simulink model "sampleModel1886"  (R2023a)
settings: Solver=VariableStepAuto  StartTime=0.0  StopTime=10.0  RelTol=1e-3
libraries: hdlsllib x5, simulink x1
settings Model: Creator=user1  LastModifiedBy=user1

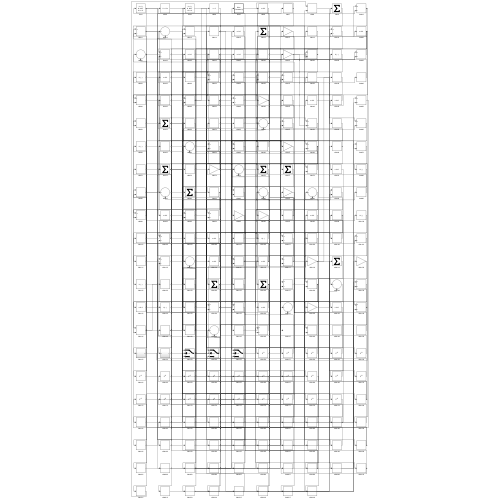
[thumbnail: Simulink's stored preview of the top-level diagram]
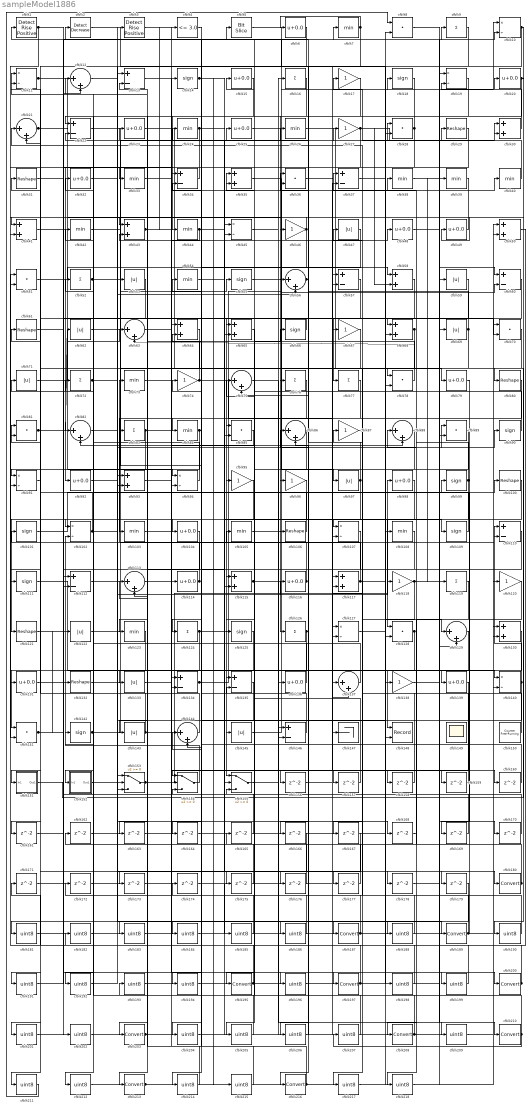
== system sampleModel1886 ==
  cfblk1 : hdlsllib/Logic and Bit Operations/Detect Rise Positive  vinit=0  OutDataTypeStr=boolean
  cfblk{10..11,19,45,91,94,102,107,127,140} (10 alike) : Product  Inputs=*/  RndMeth=Zero  SaturateOnIntegerOverflow=on
  cfblk{29,31,61,80,100,106,121,132} (8 alike) : Reshape
  cfblk{14,18,55,66,90,99,101,109,111,125,142} (11 alike) : Signum
  cfblk{7,24,26,33,38..40,42,44,54,73,84,103,105,108,123} (16 alike) : MinMax
  cfblk{6,15,20,23,25,32,48..49,79,92,98,104,114,116,131,136,139} (17 alike) : Bias  Bias=0.0  SaturateOnIntegerOverflow=off
  cfblk{13,22,34,37,57,60,110,112,134..135,146} (11 alike) : Sum  Inputs=+-
  cfblk{12,21,56,63,75,82,86,88,113,129,137,144} (12 alike) : Sum  Inputs=|++
  cfblk{30,35,41,43,50,58,64..65,68,93,115,117,130} (13 alike) : Sum
  cfblk{17,27,46,67,74,87,95..96,118,120,138} (11 alike) : Gain
  cfblk{9,16,52,72,76..77,83,119,124,126} (10 alike) : Sum  Inputs=+
  cfblk{47,53,59,62,69,71,97,122,133,143,145} (11 alike) : Abs  SaturateOnIntegerOverflow=off
  cfblk{8,28,36,51,70,78,81,85,89,128,141} (11 alike) : DotProduct  OutDataTypeStr=Inherit: Inherit via internal rule
  cfblk147 : Terminator
  cfblk148 : Record  FileSettingsInternal="{\"entries\":[{\"content\":{\"excelSettings\":{\"content\":{},\"type\":\"Streamout.ExcelSettings\"}},\"type\":\"Streamout.FileSettingStorage\",\"uuid\":\"\"}],\"packageUris\":[\"http:\\/\\/schema.mathworks.com\\/mf0\\/streamout_blocks\\/R2020a\"],\"version\":\"1.0\"}"  Layout=[1 1]  SignalsInternal="{\"entries\":[{\"content\":{\"signals\":[{\"content\":{\"blockPath\":[],\"dimensions\":[1],\"domain\":\"\",\"lineColor\":\"#a2142f\",\"plots\":[1],\"port\":1,\"signalID\":4786,\"signalName\":\"XY Graph:1\"},\"type\":\"RecordBlkView.Signal\",\"uuid\":\"\"},{\"content\":{\"blockPath\":[],\"dimensions\":[1],\"domain\":\"\",\"lineColor\":\"#139fff\",\"plots\":[1],\"port\":2,\"signalID\":4789,\"signalName\":\"XY Graph:2\"},\"type\":\"RecordBlkView.Signal\",\"uuid\":\"\"}]},\"type\":\"RecordBlkView.InputSignals\",\"uuid\":\"\"}],\"packageUris\":[\"http:\\/\\/schema.mathworks.com\\/mf0\\/streamout_blocks\\/R2020a\"],\"version\":\"1.0\"}"  VisualizationBindings="{\"xyplotplugin\":{\"info\":[{\"series\":[{\"bindingParametersList\":[{\"parameter\":\"X-Axis\",\"signalID\":4786,\"signalName\":\"XY Graph:1\"},{\"parameter\":\"Y-Axis\",\"signalID\":4789,\"signalName\":\"XY Graph:2\"}],\"seriesID\":2000}],\"subplotID\":1}]}}"  CompatibilityTag=XY  st=-1
  cfblk149 : Scope
      settings: Floating=on
  cfblk150 : hdlsllib/Sources/Counter Free-Running  NumBits=16  tsamp=-1
  cfblk151 : Subsystem
      settings: LibrarySourceBlock=|
      | hdlsllib/Ports &
      | Subsystems/Subsystem
  cfblk152 : Subsystem
      settings: LibrarySourceBlock=|
      | hdlsllib/Ports &
      | Subsystems/Subsystem
  cfblk153 : Switch  SaturateOnIntegerOverflow=off  InputSameDT=off
  cfblk154 : Switch  SaturateOnIntegerOverflow=off  InputSameDT=off
  cfblk155 : Switch  SaturateOnIntegerOverflow=off  InputSameDT=off
  cfblk{156..179} (24 alike) : Delay  SampleTime=1
  cfblk{180,187,189,195,197,200,203,208,210,213,216} (11 alike) : DataTypeConversion  SaturateOnIntegerOverflow=off  RndMeth=Floor
  cfblk{181..186,188,190..194,196,198..199,201..202,204..207,209,211..212,214..215,217..218} (28 alike) : DataTypeConversion  OutDataTypeStr=uint8  SaturateOnIntegerOverflow=off  RndMeth=Floor
  cfblk2 : simulink/Logic and Bit Operations/Detect Decrease  vinit=0.0  OutDataTypeStr=boolean
      settings: LibrarySourceBlock=|
      | hdlsllib/Logic and Bit
      | Operations/Detect
      | Decrease
  cfblk3 : hdlsllib/Logic and Bit Operations/Detect Rise Positive  vinit=0  OutDataTypeStr=boolean
  cfblk4 : hdlsllib/Logic and Bit Operations/Compare To Constant  relop=<=  const=3.0  OutDataTypeStr=boolean
  cfblk5 : hdlsllib/Logic and Bit Operations/Bit Slice  lidx=7  ridx=0
  wires:
  cfblk11/1 -> cfblk94/1, cfblk115/2
  cfblk26/1 -> cfblk79/1
  cfblk95/1 -> cfblk155/1
  cfblk62/1 -> cfblk104/1
  cfblk108/1 -> cfblk195/1
  cfblk145/1 -> cfblk7/1
  cfblk10/1 -> cfblk96/1, cfblk190/1
  cfblk69/1 -> cfblk2/1, cfblk125/1
  cfblk30/1 -> cfblk20/1
  cfblk43/1 -> cfblk4/1, cfblk158/1
  cfblk136/1 -> cfblk74/1
  cfblk132/1 -> cfblk55/1
  cfblk112/1 -> cfblk30/1
  cfblk12/1 -> cfblk189/1
  cfblk91/1 -> cfblk31/1
  cfblk116/1 -> cfblk25/1, cfblk81/2
  cfblk115/1 -> cfblk18/1, cfblk209/1
  cfblk117/1 -> cfblk73/1, cfblk129/1
  cfblk96/1 -> cfblk121/1
  cfblk39/1 -> cfblk51/2
  cfblk35/1 -> cfblk97/1
  cfblk99/1 -> cfblk37/1, cfblk154/2, cfblk111/1
  cfblk42/1 -> cfblk145/1
  cfblk134/1 -> cfblk27/1, cfblk176/1
  cfblk23/1 -> cfblk78/1
  cfblk109/1 -> cfblk5/1
  cfblk72/1 -> cfblk139/1, cfblk56/2, cfblk168/1
  cfblk77/1 -> cfblk155/2
  cfblk90/1 -> cfblk15/1
  cfblk93/1 -> cfblk114/1
  cfblk18/1 -> cfblk126/1
  cfblk51/1 -> cfblk58/1
  cfblk94/1 -> cfblk71/1
  cfblk105/1 -> cfblk100/1
  cfblk71/1 -> cfblk63/1
  cfblk5/1 -> cfblk137/2
  cfblk78/1 -> cfblk35/1
  cfblk114/1 -> cfblk21/2, cfblk81/1
  cfblk27/1 -> cfblk92/1, cfblk58/2, cfblk30/2
  cfblk101/1 -> cfblk19/1
  cfblk47/1 -> cfblk84/1
  cfblk22/1 -> cfblk147/1
  cfblk103/1 -> cfblk48/1
  cfblk76/1 -> cfblk103/1
  cfblk120/1 -> cfblk208/1
  cfblk15/1 -> cfblk44/1
  cfblk118/1 -> cfblk39/1, cfblk167/1, cfblk170/1
  cfblk1/1 -> cfblk34/1, cfblk91/2, cfblk199/1
  cfblk28/1 -> cfblk102/1, cfblk22/1
  cfblk131/1 -> cfblk102/2
  cfblk111/1 -> cfblk135/1
  cfblk54/1 -> cfblk109/1
  cfblk6/1 -> cfblk151/1(In1)
  cfblk87/1 -> cfblk187/1
  cfblk60/1 -> cfblk95/1
  cfblk64/1 -> cfblk213/1
  cfblk127/1 -> cfblk200/1
  cfblk59/1 -> cfblk85/1
  cfblk81/1 -> cfblk62/1, cfblk9/1
  cfblk130/1 -> cfblk216/1
  cfblk17/1 -> cfblk152/1(In1)
  cfblk153/1 -> cfblk98/1, cfblk40/1, cfblk178/1
  cfblk74/1 -> cfblk117/2, cfblk11/2, cfblk106/1
  cfblk133/1 -> cfblk14/1
  cfblk142/1 -> cfblk110/1, cfblk118/1
  cfblk124/1 -> cfblk37/2, cfblk133/1
  cfblk102/1 -> cfblk61/1, cfblk89/1
  cfblk84/1 -> cfblk24/1, cfblk131/1
  cfblk52/1 -> cfblk77/1, cfblk148/2
  cfblk144/1 -> cfblk101/1
  cfblk98/1 -> cfblk128/1
  cfblk150/1 -> cfblk47/1
  cfblk58/1 -> cfblk143/1
  cfblk20/1 -> cfblk49/1, cfblk56/1, cfblk19/2, cfblk28/2
  cfblk126/1 -> cfblk163/1, cfblk206/1
  cfblk41/1 -> cfblk67/1
  cfblk128/1 -> cfblk148/1, cfblk141/1
  cfblk73/1 -> cfblk76/1
  cfblk53/1 -> cfblk91/1
  cfblk21/1 -> cfblk46/1, cfblk211/1
  cfblk137/1 -> cfblk42/1
  cfblk113/1 -> cfblk105/1
  cfblk16/1 -> cfblk203/1
  cfblk3/1 -> cfblk180/1
  cfblk139/1 -> cfblk154/1
  cfblk2/1 -> cfblk138/1
  cfblk140/1 -> cfblk110/2, cfblk144/2
  cfblk40/1 -> cfblk17/1
  cfblk13/1 -> cfblk197/1
  cfblk83/1 -> cfblk66/1, cfblk28/1, cfblk141/2
  cfblk24/1 -> cfblk140/1, cfblk124/1, cfblk41/2
  cfblk154/1 -> cfblk132/1
  cfblk61/1 -> cfblk68/1
  cfblk56/1 -> cfblk36/1, cfblk36/2
  cfblk82/1 -> cfblk53/1
  cfblk7/1 -> cfblk6/1, cfblk93/2
  cfblk67/1 -> cfblk83/1
  cfblk48/1 -> cfblk60/1
  cfblk88/1 -> cfblk146/2
  cfblk146/1 -> cfblk54/1
  cfblk141/1 -> cfblk112/2, cfblk122/1
  cfblk151/1(Out1) -> cfblk80/1
  cfblk75/1 -> cfblk136/1
  cfblk45/1 -> cfblk29/1
  cfblk122/1 -> cfblk116/1
  cfblk85/1 -> cfblk82/2
  cfblk25/1 -> cfblk10/1
  cfblk68/1 -> cfblk63/2, cfblk107/1, cfblk212/1
  cfblk106/1 -> cfblk52/1
  cfblk34/1 -> cfblk33/1
  cfblk33/1 -> cfblk88/2
  cfblk49/1 -> cfblk43/1
  cfblk9/1 -> cfblk134/2
  cfblk65/1 -> cfblk115/1
  cfblk143/1 -> cfblk72/1, cfblk90/1, cfblk11/1
  cfblk138/1 -> cfblk10/2
  cfblk8/1 -> cfblk210/1
  cfblk14/1 -> cfblk70/2, cfblk215/1
  cfblk19/1 -> cfblk123/1
  cfblk46/1 -> cfblk85/2, cfblk41/1
  cfblk38/1 -> cfblk59/1
  cfblk97/1 -> cfblk75/2, cfblk113/2, cfblk22/2
  cfblk55/1 -> cfblk60/2
  cfblk66/1 -> cfblk65/1
  cfblk44/1 -> cfblk26/1, cfblk43/2
  cfblk29/1 -> cfblk65/2
  cfblk80/1 -> cfblk156/1
  cfblk156/1 -> cfblk137/1
  cfblk155/1 -> cfblk157/1
  cfblk157/1 -> cfblk75/1
  cfblk158/1 -> cfblk21/1
  cfblk63/1 -> cfblk159/1
  cfblk159/1 -> cfblk117/1
  cfblk36/1 -> cfblk160/1
  cfblk160/1 -> cfblk1/1
  cfblk123/1 -> cfblk161/1
  cfblk161/1 -> cfblk82/1
  cfblk162/1 -> cfblk128/2
  cfblk163/1 -> cfblk68/2
  cfblk135/1 -> cfblk164/1
  cfblk164/1 -> cfblk78/2
  cfblk165/1 -> cfblk112/1
  cfblk110/1 -> cfblk166/1
  cfblk79/1 -> cfblk169/1
  cfblk169/1 -> cfblk88/1
  cfblk170/1 -> cfblk153/2
  cfblk171/1 -> cfblk153/3
  cfblk172/1 -> cfblk107/2
  cfblk125/1 -> cfblk173/1
  cfblk173/1 -> cfblk146/1
  cfblk92/1 -> cfblk175/1
  cfblk175/1 -> cfblk134/1
  cfblk176/1 -> cfblk93/1
  cfblk152/1(Out1) -> cfblk177/1
  cfblk177/1 -> cfblk35/2
  cfblk178/1 -> cfblk129/2
  cfblk32/1 -> cfblk179/1
  cfblk180/1 -> cfblk38/1, cfblk32/1
  cfblk179/1 -> cfblk181/1
  cfblk181/1 -> cfblk3/1
  cfblk50/1 -> cfblk182/1
  cfblk182/1 -> cfblk94/2
  cfblk104/1 -> cfblk183/1
  cfblk183/1 -> cfblk50/1
  cfblk4/1 -> cfblk184/1
  cfblk184/1 -> cfblk50/2
  cfblk174/1 -> cfblk185/1
  cfblk185/1 -> cfblk34/2
  cfblk89/1 -> cfblk186/1
  cfblk186/1 -> cfblk174/1
  cfblk187/1 -> cfblk165/1, cfblk142/1
  cfblk119/1 -> cfblk188/1
  cfblk188/1 -> cfblk87/1
  cfblk189/1 -> cfblk144/1, cfblk99/1
  cfblk190/1 -> cfblk12/1
  cfblk70/1 -> cfblk191/1
  cfblk191/1 -> cfblk12/2
  cfblk57/1 -> cfblk192/1
  cfblk192/1 -> cfblk153/1
  cfblk193/1 -> cfblk57/1
  cfblk166/1 -> cfblk194/1
  cfblk194/1 -> cfblk57/2
  cfblk195/1 -> cfblk172/1, cfblk51/1
  cfblk121/1 -> cfblk196/1
  cfblk196/1 -> cfblk108/1
  cfblk197/1 -> cfblk171/1, cfblk119/1
  cfblk37/1 -> cfblk198/1
  cfblk198/1 -> cfblk13/1
  cfblk199/1 -> cfblk13/2
  cfblk200/1 -> cfblk154/3, cfblk23/1
  cfblk167/1 -> cfblk201/1
  cfblk201/1 -> cfblk127/1
  cfblk31/1 -> cfblk202/1
  cfblk202/1 -> cfblk127/2
  cfblk203/1 -> cfblk70/1, cfblk45/2, cfblk45/1
  cfblk100/1 -> cfblk204/1
  cfblk204/1 -> cfblk16/1
  cfblk86/1 -> cfblk205/1
  cfblk205/1 -> cfblk162/1
  cfblk206/1 -> cfblk86/1
  cfblk207/1 -> cfblk86/2
  cfblk208/1 -> cfblk135/2, cfblk155/3
  cfblk209/1 -> cfblk120/1
  cfblk210/1 -> cfblk207/1, cfblk113/1
  cfblk211/1 -> cfblk8/1
  cfblk212/1 -> cfblk8/2
  cfblk213/1 -> cfblk140/2, cfblk69/1
  cfblk107/1 -> cfblk214/1
  cfblk214/1 -> cfblk64/1
  cfblk215/1 -> cfblk64/2
  cfblk216/1 -> cfblk193/1, cfblk89/2
  cfblk129/1 -> cfblk217/1
  cfblk217/1 -> cfblk130/1
  cfblk168/1 -> cfblk218/1
  cfblk218/1 -> cfblk130/2

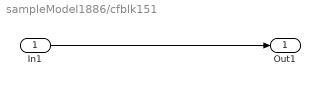
== system sampleModel1886/cfblk151 ==
  In1 : Inport
  Out1 : Outport
  wires:
  In1/1 -> Out1/1

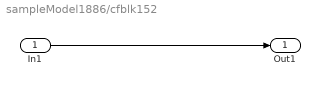
== system sampleModel1886/cfblk152 ==
  In1 : Inport
  Out1 : Outport
  wires:
  In1/1 -> Out1/1
